simulink model "controller_sim6"  (Simulink 7.7)
settings: Solver=ode45  StartTime=0.0  StopTime=0.9  RelTol=1e-3
libraries: simulink x2
settings Model: Creator=Mikael  LastModifiedBy=Mikael
settings DataIOCC: LimitDataPoints=off

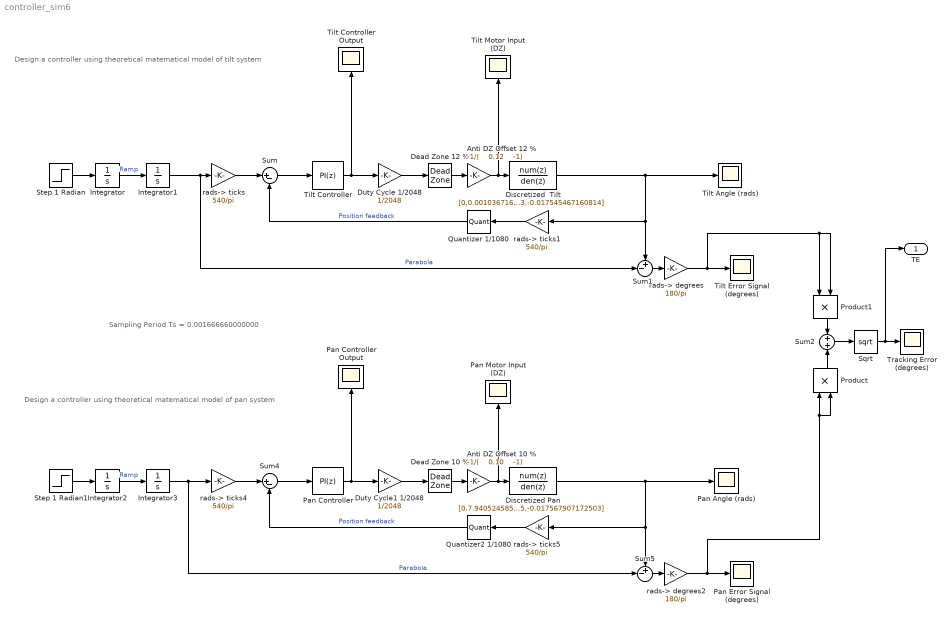
== system controller_sim6 ==
  note: Design a controller
      | using theoretical matematical
      | model of tilt system
  note: Design a controller
      | using theoretical matematical
      | model of pan system
  note: Sampling Period
      | Ts = 0.001666660000000
  Anti DZ Offset 10 % : Gain  Gain="-1/(    0.10    -1)"
  Anti DZ Offset 12 % : Gain  Gain="-1/(    0.12    -1)"
  Dead Zone 10 % : DeadZone  LowerValue=-0.10  UpperValue=0.10  SaturateOnIntegerOverflow=on
  Dead Zone 12 % : DeadZone  LowerValue=-0.12  UpperValue=0.12  SaturateOnIntegerOverflow=on
  Discretized Pan : DiscreteTransferFcn  Numerator=[0,7.940524585890426e-04,0.001559625676259,1.183839817575144e-04]  Denominator=[1,-1.949665306697232,0.967233213869735,-0.017567907172503]  SampleTime=0.001666660000000
  Discretized  Tilt : DiscreteTransferFcn  Numerator=[0,0.001036716194946,0.002027296745175,1.540816979825817e-04]  Denominator=[1,-1.929150845911249,0.946696313072063,-0.017545467160814]  SampleTime=0.001666660000000
  Duty Cycle 1/2048 : Gain  Gain=1/2048
  Duty Cycle1 1/2048 : Gain  Gain=1/2048
  Integrator{,1..3} (4 alike) : Integrator
  Pan Angle (rads) : Scope
      settings: SaveName=ScopeData6
  Pan Controller : simulink/Continuous/PID Controller  SystemSampleTime=-1  Controller=PI  TimeDomain=Discrete-time  SampleTime=0.001666660000000  IntegratorMethod=Forward Euler  FilterMethod=Forward Euler  Form=Parallel  P=240  I=100  D=2  N=1  InitialConditionSource=internal  InitialConditionForIntegrator=0  InitialConditionForFilter=0  ExternalReset=none  LimitOutput=on  UpperSaturationLimit=2047  LowerSaturationLimit=-2047  LinearizeAsGain=off  AntiWindupMode=none  Kb=1  TrackingMode=off  Kt=1  PParamMin=[]  PParamMax=[]  IParamMin=[]  IParamMax=[]  DParamMin=[]  DParamMax=[]  NParamMin=[]  NParamMax=[]  KbParamMin=[]  KbParamMax=[]  KtParamMin=[]  KtParamMax=[]  POutMin=[]  POutMax=[]  IOutMin=[]  IOutMax=[]  DOutMin=[]  DOutMax=[]  NOutMin=[]  NOutMax=[]  KbOutMin=[]  KbOutMax=[]  KtOutMin=[]  KtOutMax=[]  IntegratorOutMin=[]  IntegratorOutMax=[]  FilterOutMin=[]  FilterOutMax=[]  SumOutMin=[]  SumOutMax=[]  SumI1OutMin=[]  SumI1OutMax=[]  SumI2OutMin=[]  SumI2OutMax=[]  SumI3OutMin=[]  SumI3OutMax=[]  SumDOutMin=[]  SumDOutMax=[]  SaturationOutMin=[]  SaturationOutMax=[]  IntegratorContinuousStateAttributes=''  IntegratorStateMustResolveToSignalObject=off  IntegratorRTWStateStorageClass=Auto  FilterContinuousStateAttributes=''  FilterStateMustResolveToSignalObject=off  FilterRTWStateStorageClass=Auto
  Pan Error Signal (degrees) : Scope
      settings: SaveName=ScopeData4
  Pan Controller Output : Scope
      settings: SaveName=ScopeData5
  Pan Motor Input (DZ) : Scope
      settings: SaveName=ScopeData7
  Product : Product  RndMeth=Zero
  Product1 : Product  RndMeth=Zero
  Quantizer 1/1080 : Quantizer  QuantizationInterval=1/1080  SampleTime=0.00166666000000
  Quantizer2 1/1080 : Quantizer  QuantizationInterval=1/1080  SampleTime=0.00166666000000
  Sqrt : Sqrt  SaturateOnIntegerOverflow=on
  Step 1 Radian : Step  Time=0  SampleTime=0
  Step 1 Radian1 : Step  Time=0  SampleTime=0
  Sum : Sum  Inputs=|+-
  Sum1 : Sum  Inputs=+-|
  Sum2 : Sum  Inputs=+|+
  Sum4 : Sum  Inputs=|+-
  Sum5 : Sum  Inputs=+-|
  Tilt Angle (rads) : Scope
  Tilt Controller : simulink/Continuous/PID Controller  SystemSampleTime=-1  Controller=PI  TimeDomain=Discrete-time  SampleTime=0.001666660000000  IntegratorMethod=Forward Euler  FilterMethod=Forward Euler  Form=Parallel  P=240  I=85  D=2  N=1  InitialConditionSource=internal  InitialConditionForIntegrator=0  InitialConditionForFilter=0  ExternalReset=none  LimitOutput=on  UpperSaturationLimit=2047  LowerSaturationLimit=-2047  LinearizeAsGain=off  AntiWindupMode=none  Kb=1  TrackingMode=off  Kt=1  PParamMin=[]  PParamMax=[]  IParamMin=[]  IParamMax=[]  DParamMin=[]  DParamMax=[]  NParamMin=[]  NParamMax=[]  KbParamMin=[]  KbParamMax=[]  KtParamMin=[]  KtParamMax=[]  POutMin=[]  POutMax=[]  IOutMin=[]  IOutMax=[]  DOutMin=[]  DOutMax=[]  NOutMin=[]  NOutMax=[]  KbOutMin=[]  KbOutMax=[]  KtOutMin=[]  KtOutMax=[]  IntegratorOutMin=[]  IntegratorOutMax=[]  FilterOutMin=[]  FilterOutMax=[]  SumOutMin=[]  SumOutMax=[]  SumI1OutMin=[]  SumI1OutMax=[]  SumI2OutMin=[]  SumI2OutMax=[]  SumI3OutMin=[]  SumI3OutMax=[]  SumDOutMin=[]  SumDOutMax=[]  SaturationOutMin=[]  SaturationOutMax=[]  IntegratorContinuousStateAttributes=''  IntegratorStateMustResolveToSignalObject=off  IntegratorRTWStateStorageClass=Auto  FilterContinuousStateAttributes=''  FilterStateMustResolveToSignalObject=off  FilterRTWStateStorageClass=Auto
  Tilt Error Signal (degrees) : Scope
      settings: SaveName=ScopeData3
  Tilt Controller Output : Scope
  Tilt Motor Input (DZ) : Scope
      settings: SaveName=ScopeData2
  Tracking Error (degrees) : Scope
      settings: TimeRange=0.9  YMin=0  YMax=1  SaveName=ScopeData8
  rads-> degrees : Gain  Gain=180/pi
  rads-> degrees2 : Gain  Gain=180/pi
  rads-> ticks{,1,4..5} (4 alike) : Gain  Gain=540/pi
  TE : Outport
  wires:
  Step 1 Radian/1 -> Integrator/1
  Sum/1 -> Tilt Controller/1
  Tilt Controller/1 -> Tilt Controller Output/1, Duty Cycle 1/2048/1
  Discretized  Tilt/1 -> rads-> ticks1/1, Sum1/1, Tilt Angle (rads)/1
  Dead Zone 12 %/1 -> Anti DZ Offset 12 %/1
  Anti DZ Offset 12 %/1 -> Discretized  Tilt/1, Tilt Motor Input (DZ)/1
  Quantizer 1/1080/1 -> Sum/2  "Position feedback"
  rads-> ticks1/1 -> Quantizer 1/1080/1
  rads-> ticks/1 -> Sum/1
  rads-> degrees/1 -> Tilt Error Signal (degrees)/1, Product1/1, Product1/2
  Sum1/1 -> rads-> degrees/1
  Sum4/1 -> Pan Controller/1
  Pan Controller/1 -> Pan Controller Output/1, Duty Cycle1 1/2048/1
  Discretized Pan/1 -> rads-> ticks5/1, Sum5/1, Pan Angle (rads)/1
  Dead Zone 10 %/1 -> Anti DZ Offset 10 %/1
  Anti DZ Offset 10 %/1 -> Discretized Pan/1, Pan Motor Input (DZ)/1
  Quantizer2 1/1080/1 -> Sum4/2  "Position feedback"
  rads-> ticks5/1 -> Quantizer2 1/1080/1
  rads-> ticks4/1 -> Sum4/1
  rads-> degrees2/1 -> Pan Error Signal (degrees)/1, Product/1, Product/2
  Sum5/1 -> rads-> degrees2/1
  Duty Cycle1 1/2048/1 -> Dead Zone 10 %/1
  Duty Cycle 1/2048/1 -> Dead Zone 12 %/1
  Integrator/1 -> Integrator1/1  "Ramp"
  Integrator1/1 -> rads-> ticks/1, Sum1/2  "Parabola"
  Step 1 Radian1/1 -> Integrator2/1
  Integrator2/1 -> Integrator3/1  "Ramp"
  Integrator3/1 -> rads-> ticks4/1, Sum5/2  "Parabola"
  Product1/1 -> Sum2/1
  Product/1 -> Sum2/2
  Sum2/1 -> Sqrt/1
  Sqrt/1 -> Tracking Error (degrees)/1, TE/1
